simulink model "C_p"  (R2014a)
settings: Solver=ode3  StartTime=0.0  StopTime=0.04  FixedStep=1e-6  MaxStep=0.001  MinStep=0.0001  RelTol=1e-3
settings Model: Creator=User  LastModifiedBy=Анастасия

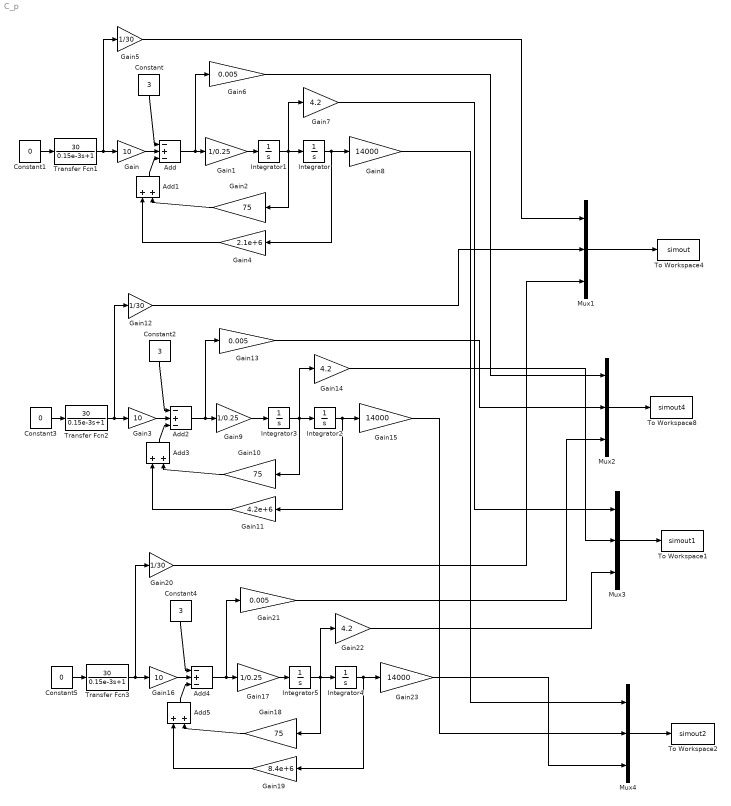
== system C_p ==
  Add : Sum  Inputs=-+-
  Add1 : Sum
  Add2 : Sum  Inputs=-+-
  Add3 : Sum
  Add4 : Sum  Inputs=-+-
  Add5 : Sum
  Constant : Constant  Value=3
  Constant1 : Constant  Value=0
  Constant2 : Constant  Value=3
  Constant3 : Constant  Value=0
  Constant4 : Constant  Value=3
  Constant5 : Constant  Value=0
  Gain : Gain  Gain=10
  Gain1 : Gain  Gain=1/0.25
  Gain10 : Gain  Gain=75
  Gain11 : Gain  Gain=4.2e+6
  Gain12 : Gain  Gain=1/30
  Gain13 : Gain  Gain=0.005
  Gain14 : Gain  Gain=4.2
  Gain15 : Gain  Gain=14000
  Gain16 : Gain  Gain=10
  Gain17 : Gain  Gain=1/0.25
  Gain18 : Gain  Gain=75
  Gain19 : Gain  Gain=8.4e+6
  Gain2 : Gain  Gain=75
  Gain20 : Gain  Gain=1/30
  Gain21 : Gain  Gain=0.005
  Gain22 : Gain  Gain=4.2
  Gain23 : Gain  Gain=14000
  Gain3 : Gain  Gain=10
  Gain4 : Gain  Gain=2.1e+6
  Gain5 : Gain  Gain=1/30
  Gain6 : Gain  Gain=0.005
  Gain7 : Gain  Gain=4.2
  Gain8 : Gain  Gain=14000
  Gain9 : Gain  Gain=1/0.25
  Integrator{,1..5} (6 alike) : Integrator
  Mux{1..4} (4 alike) : Mux  Inputs=3
  To Workspace1 : ToWorkspace  VariableName=simout1  SaveFormat=Timeseries  SampleTime=-1
  To Workspace2 : ToWorkspace  VariableName=simout2  SaveFormat=Timeseries  SampleTime=-1
  To Workspace4 : ToWorkspace  VariableName=simout  SaveFormat=Timeseries  SampleTime=-1
  To Workspace8 : ToWorkspace  VariableName=simout4  SaveFormat=Timeseries  SampleTime=-1
  Transfer Fcn1 : TransferFcn  Numerator=[30]  Denominator=[0.15e-3 1]
  Transfer Fcn2 : TransferFcn  Numerator=[30]  Denominator=[0.15e-3 1]
  Transfer Fcn3 : TransferFcn  Numerator=[30]  Denominator=[0.15e-3 1]
  wires:
  Constant1/1 -> Transfer Fcn1/1
  Transfer Fcn1/1 -> Gain/1, Gain5/1
  Integrator1/1 -> Integrator/1, Gain2/1, Gain7/1
  Integrator/1 -> Gain8/1, Gain4/1
  Gain8/1 -> Mux4/1
  Gain7/1 -> Mux3/1
  Gain6/1 -> Mux2/1
  Gain5/1 -> Mux1/1
  Gain/1 -> Add/2
  Add1/1 -> Add/3
  Add/1 -> Gain6/1, Gain1/1
  Constant/1 -> Add/1
  Gain1/1 -> Integrator1/1
  Gain2/1 -> Add1/2
  Gain4/1 -> Add1/1
  Constant3/1 -> Transfer Fcn2/1
  Transfer Fcn2/1 -> Gain3/1, Gain12/1
  Integrator3/1 -> Integrator2/1, Gain10/1, Gain14/1
  Integrator2/1 -> Gain15/1, Gain11/1
  Gain15/1 -> Mux4/2
  Gain14/1 -> Mux3/2
  Gain13/1 -> Mux2/2
  Gain12/1 -> Mux1/2
  Gain3/1 -> Add2/2
  Add3/1 -> Add2/3
  Add2/1 -> Gain13/1, Gain9/1
  Constant2/1 -> Add2/1
  Gain9/1 -> Integrator3/1
  Gain10/1 -> Add3/2
  Gain11/1 -> Add3/1
  Constant5/1 -> Transfer Fcn3/1
  Transfer Fcn3/1 -> Gain16/1, Gain20/1
  Integrator5/1 -> Integrator4/1, Gain18/1, Gain22/1
  Integrator4/1 -> Gain23/1, Gain19/1
  Gain23/1 -> Mux4/3
  Gain22/1 -> Mux3/3
  Gain21/1 -> Mux2/3
  Gain20/1 -> Mux1/3
  Gain16/1 -> Add4/2
  Add5/1 -> Add4/3
  Add4/1 -> Gain21/1, Gain17/1
  Constant4/1 -> Add4/1
  Gain17/1 -> Integrator5/1
  Gain18/1 -> Add5/2
  Gain19/1 -> Add5/1
  Mux1/1 -> To Workspace4/1
  Mux2/1 -> To Workspace8/1
  Mux3/1 -> To Workspace1/1
  Mux4/1 -> To Workspace2/1
